simulink model "E5_G1"  (R2021b)
settings: Solver=VariableStepAuto  StartTime=0.0  StopTime=1  RelTol=1e-3
settings Model: Creator=new  LastModifiedBy=new

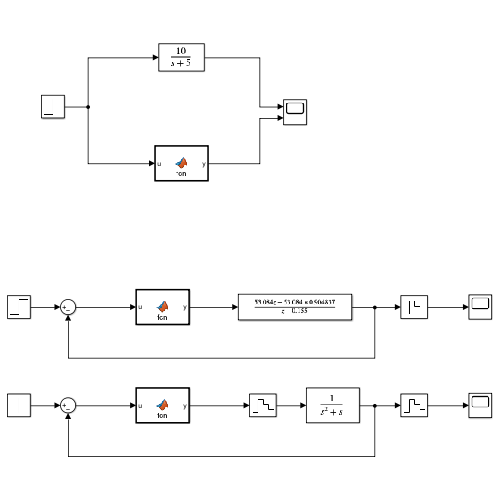
[thumbnail: Simulink's stored preview of the top-level diagram]
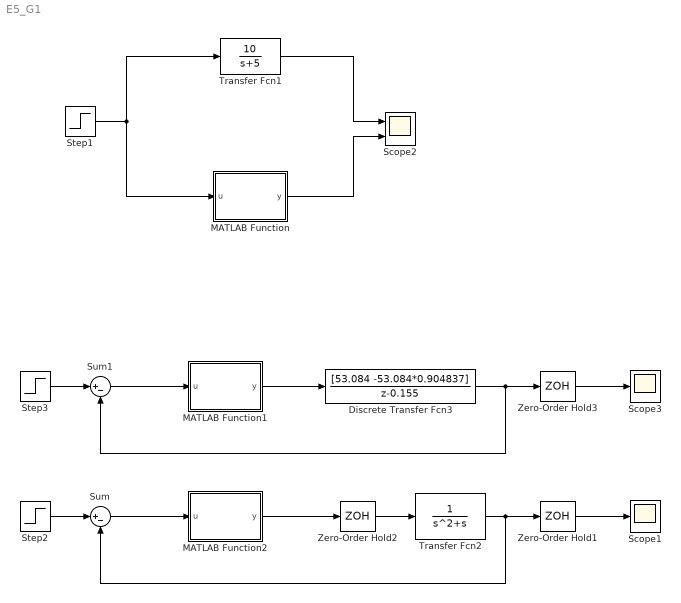
== system E5_G1 ==
  Discrete Transfer Fcn3 : DiscreteTransferFcn  Numerator=[53.084 -53.084*0.904837]  Denominator=[1 -0.155]  SampleTime=0.1
  MATLAB Function : MATLAB Function  TreatAsAtomicUnit=on  SystemSampleTime=0.04
  MATLAB Function1 : MATLAB Function  TreatAsAtomicUnit=on  SystemSampleTime=0.04
  MATLAB Function2 : MATLAB Function  TreatAsAtomicUnit=on  SystemSampleTime=0.04
  Scope1 : Scope
  Scope2 : Scope  NumInputPorts=2
  Scope3 : Scope
  Step1 : Step  Time=0  SampleTime=0
  Step2 : Step  SampleTime=0
  Step3 : Step  SampleTime=0
  Sum : Sum  Inputs=|+-
  Sum1 : Sum  Inputs=|+-
  Transfer Fcn1 : TransferFcn  Numerator=[10]  Denominator=[1 5]
  Transfer Fcn2 : TransferFcn  Denominator=[1 1 0]
  Zero-Order Hold1 : ZeroOrderHold  SampleTime=0.1
  Zero-Order Hold2 : ZeroOrderHold  SampleTime=0.1
  Zero-Order Hold3 : ZeroOrderHold  SampleTime=0.1
  wires:
  Transfer Fcn1/1 -> Scope2/1
  Step1/1 -> MATLAB Function/1(u), Transfer Fcn1/1
  MATLAB Function/1(y) -> Scope2/2
  Zero-Order Hold1/1 -> Scope1/1
  Transfer Fcn2/1 -> Sum/2, Zero-Order Hold1/1
  Zero-Order Hold2/1 -> Transfer Fcn2/1
  MATLAB Function2/1(y) -> Zero-Order Hold2/1
  Sum/1 -> MATLAB Function2/1(u)
  Step2/1 -> Sum/1
  Step3/1 -> Sum1/1
  Sum1/1 -> MATLAB Function1/1(u)
  Discrete Transfer Fcn3/1 -> Zero-Order Hold3/1, Sum1/2
  Zero-Order Hold3/1 -> Scope3/1
  MATLAB Function1/1(y) -> Discrete Transfer Fcn3/1

== matlab function E5_G1/MATLAB Function ==
  data: u input; y output
function y = fcn(u)
    persistent u0 u1 y0 y1
    
    if isempty(u0)
        u1=0;u0=0;y1=0;y0=0;
    end
    
    u1=u0;y1=y0;
    u0=u;
    y=0.36254*u1+0.8187*y1;
    y0=y;

== matlab function E5_G1/MATLAB Function2 ==
  data: u input; y output
function y = fcn(u)
    persistent u0 u1 y0 y1
    
    if isempty(u0)
        u1=0;u0=0;y1=0;y0=0;
    end
    
    u1=u0;y1=y0;
    u0=u;
    y=0.36254*u1+0.8187*y1;
    y0=y;

== matlab function E5_G1/MATLAB Function1 ==
  data: u input; y output
function y = fcn(u)
